simulink model "AM"  (R2024b)
settings: Solver=VariableStepAuto  StartTime=0.0  StopTime=0.001  RelTol=1e-3  EnableMultiTasking=on
settings Model: Creator=Usuario  LastModifiedBy=RomaW11
settings SolverCC: AlgebraicLoopSolver=TrustRegion
settings DataIOCC: LimitDataPoints=on  ReturnWorkspaceOutputs=off
settings OptimizationCC: LifeSpan=inf
settings DebuggingCC: UnconnectedInputMsg=warning  UnconnectedOutputMsg=warning  UnconnectedLineMsg=warning  AllowSymbolicDim=off  SFUnexpectedBacktrackingDiag=warning  SFNoUnconditionalDefaultTransitionDiag=warning  SFExecutionAtInitializationDiag=none  ArithmeticOperatorsInVariantConditions=warning
settings ModelReferenceCC: EnableRefExpFcnMdlSchedulingChecks=on  PropagateSignalLabelsOutOfModel=off
settings SFSimCC: SimUseLocalCustomCode=off  CustomCodeUndefinedFunction=UseInterfaceOnly
settings RTWCC: RTWUseLocalCustomCode=off  GPUComputeCapability=3.5
settings CodeAppCC: StateflowObjectComments=on
settings GRTTargetCC: TargetLangStandard=C89/C90 (ANSI)
settings ConfigComp: CovMetricSettings=dw  CovSaveCumulativeToWorkspaceVar=on  CovSaveSingleToWorkspaceVar=on  CovExternalEMLEnable=off

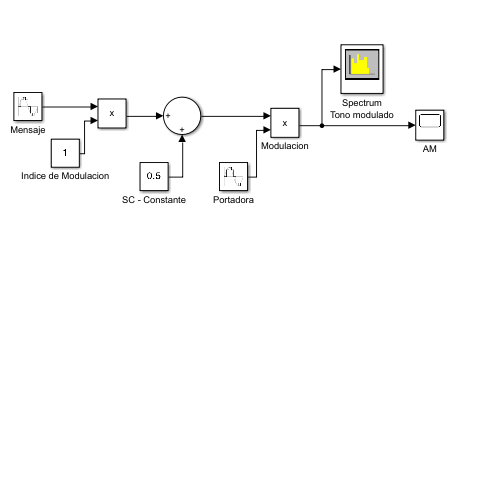
[thumbnail: Simulink's stored preview of the top-level diagram]
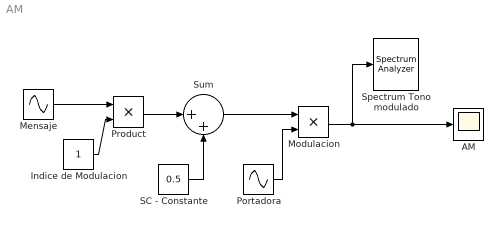
== system AM ==
  AM : Scope
  Indice de Modulacion : Constant
  Mensaje : Sin  Frequency=2*pi*1e6  SampleTime=1/(1e9)
  "Modulacion " : Product
  "Portadora " : Sin  Frequency=2*pi*(10e6)  SampleTime=1/(1e9)
  Product : Product
  SC - Constante : Constant  Value=0.5
  Spectrum Tono modulado : SpectrumAnalyzer  WindowPosition=[-958.000000,-5.000000,958.000000,1048.000000,]  ScopeFrameLocation=window  Method=Welch  SampleRate=1000000000  AxesScaling=Manual  FrequencySpan=Span and center frequency  Span=5e6  CenterFrequency=10e6  StartFrequency=-500000000  StopFrequency=500000000  AveragingMethod=Running  YLabel=dBm  YLimits=[-137.9101002091548,88.02942452262732]  ShowGrid=off  SelectedToolstripTab=spectrumAnalyzerToolstrip.measurementsTab  AllowFFTLengthLessThanSamplesPerUpdate=on  DefaultConfigurationName=spbscopes.SpectrumAnalyzerBlockCfg
  Sum : Sum  Inputs=|++
  wires:
  SC - Constante/1 -> Sum/2
  Mensaje/1 -> Product/1
  Product/1 -> Sum/1
  Indice de Modulacion/1 -> Product/2
  Sum/1 -> "Modulacion "/1
  "Portadora "/1 -> "Modulacion "/2
  "Modulacion "/1 -> Spectrum Tono modulado/1, AM/1
